simulink model "planGlobal_sim"  (R2024b)
settings: Solver=VariableStepAuto  StartTime=0.0  StopTime=10.0  RelTol=1e-3
InitFcn:
  | globalPlanSetup
undefined symbols (not defined in the file): dem, goal, gridLoc, res, start, tuneableTerrainAwareParams
libraries: roshelperlib x2, simulink x1
settings Model: Creator=cstabile  LastModifiedBy=jbrault
settings SolverCC: DateTimeAtSimulationTimeZero=[]

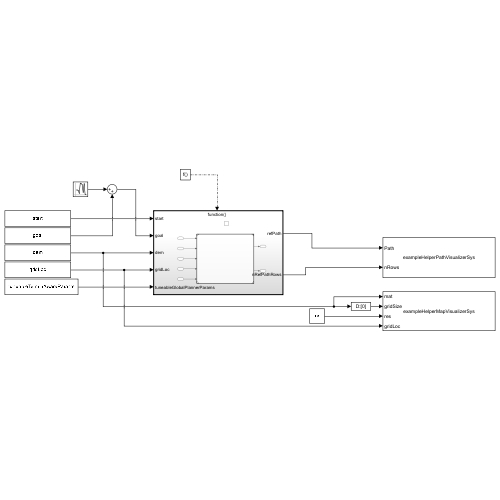
[thumbnail: Simulink's stored preview of the top-level diagram]
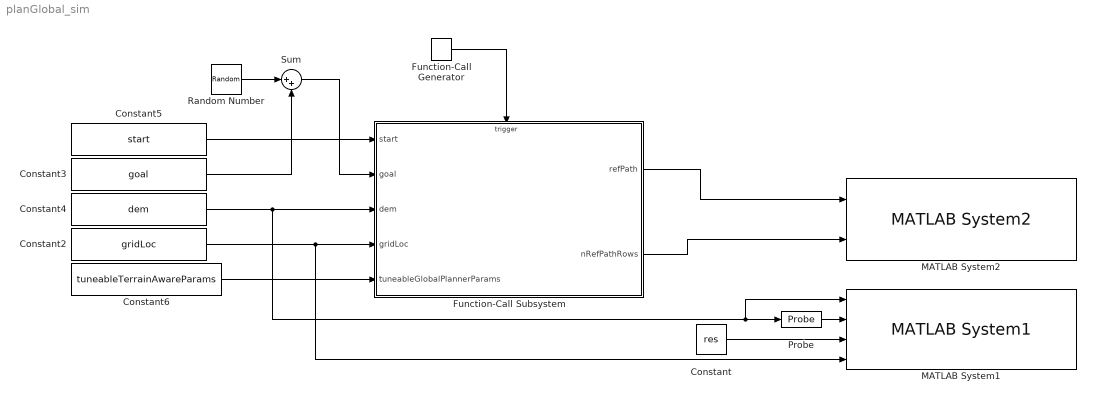
== system planGlobal_sim ==
  Constant : Constant  Value=res
  Constant2 : Constant  Value=gridLoc
  Constant3 : Constant  Value=goal
  Constant4 : Constant  Value=dem
  Constant5 : Constant  Value=start
  Constant6 : Constant  Value=tuneableTerrainAwareParams  OutDataTypeStr=Bus: fsp_tunable_bus
  Function-Call Generator : simulink/Ports & Subsystems/Function-Call Generator  sample_time=1  numberOfIterations=1  DisallowWideOutput=off
  Function-Call Subsystem : Subsystem  TreatAsAtomicUnit=on
  MATLAB System1 : roshelperlib/MATLAB System1  MapType=Generic  IsEgo=off  DisplayVisual=on  SimulateUsing=Interpreted execution
  MATLAB System2 : roshelperlib/MATLAB System2  VisualizationParameters={'k-'}  PlotType=Line  DisplayVisual=on  SimulateUsing=Interpreted execution
  Probe : Probe  ProbeWidth=off  ProbeSampleTime=off  ProbeComplexSignal=off  ProbeSignalDimensions=on
  Random Number : RandomNumber  Mean=[0 0 0]  Variance=10  SampleTime=0.1
  Sum : Sum  Inputs=|++
  wires:
  Function-Call Generator/1 -> Function-Call Subsystem/Trigger
  Constant2/1 -> MATLAB System1/4, Function-Call Subsystem/4(gridLoc)
  Constant4/1 -> MATLAB System1/1, Probe/1, Function-Call Subsystem/3(dem)
  Constant5/1 -> Function-Call Subsystem/1(start)
  Constant3/1 -> Sum/2
  Constant6/1 -> Function-Call Subsystem/5(tuneableGlobalPlannerParams)
  Function-Call Subsystem/1(refPath) -> MATLAB System2/1
  Function-Call Subsystem/2(nRefPathRows) -> MATLAB System2/2
  Constant/1 -> MATLAB System1/3
  Probe/1 -> MATLAB System1/2
  Random Number/1 -> Sum/1
  Sum/1 -> Function-Call Subsystem/2(goal)

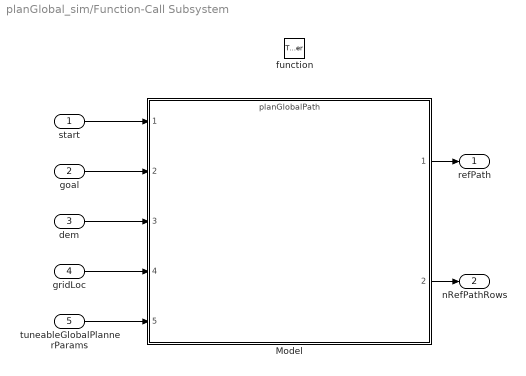
== system planGlobal_sim/Function-Call Subsystem ==
  start : Inport
  goal : Inport  Port=2
  dem : Inport  Port=3
  gridLoc : Inport  Port=4
  tuneableGlobalPlannerParams : Inport  Port=5  OutDataTypeStr=Bus: fsp_tunable_bus
  function : TriggerPort  TriggerType=function-call  VariantControl=(inherit)
  Model : ModelReference  ModelNameDialog=planGlobalPath.slx  SimulationMode=Normal  ModelReferenceVersion=2.0
  refPath : Outport
  nRefPathRows : Outport  Port=2
  wires:
  Model/2 -> nRefPathRows/1
  start/1 -> Model/1
  dem/1 -> Model/3
  goal/1 -> Model/2
  gridLoc/1 -> Model/4
  Model/1 -> refPath/1
  tuneableGlobalPlannerParams/1 -> Model/5
